simulink model "swing_up_sim"  (R2021a)
settings: Solver=VariableStepAuto  StartTime=0.0  StopTime=Inf  RelTol=1e-3
values from neighbouring files (symbols this model uses):
  alpha_0 = 0.0*pi    (= 0)    [swing_up_simulator.m]
  bp = 5e-5    (= 5e-05)    [qube2_rotpen_param.m]
  br = 1e-3    (= 0.001)    [qube2_rotpen_param.m]
  g = 9.81    [qube2_rotpen_param.m]
  Jp = mp*Lp^2/3    (= 0.000133128)    [qube2_rotpen_param.m]
  Jr = mr*r^2/3    (= 0.000228791666667)    [qube2_rotpen_param.m]
  l = Lp/2    (= 0.0645)    [qube2_rotpen_param.m]
  mp = 0.024    [qube2_rotpen_param.m]
  r = 0.085    [qube2_rotpen_param.m]
  tau_max = kt*10/Rm    (= 0.05)    [qube2_rotpen_param.m]
  thetadd_max = a_max/r    (= 72.8464760517)    [qube2_rotpen_param.m]
undefined symbols (not defined in the file or in its folder): rl
libraries: rllib x1
settings Model: Creator=willi  LastModifiedBy=willi

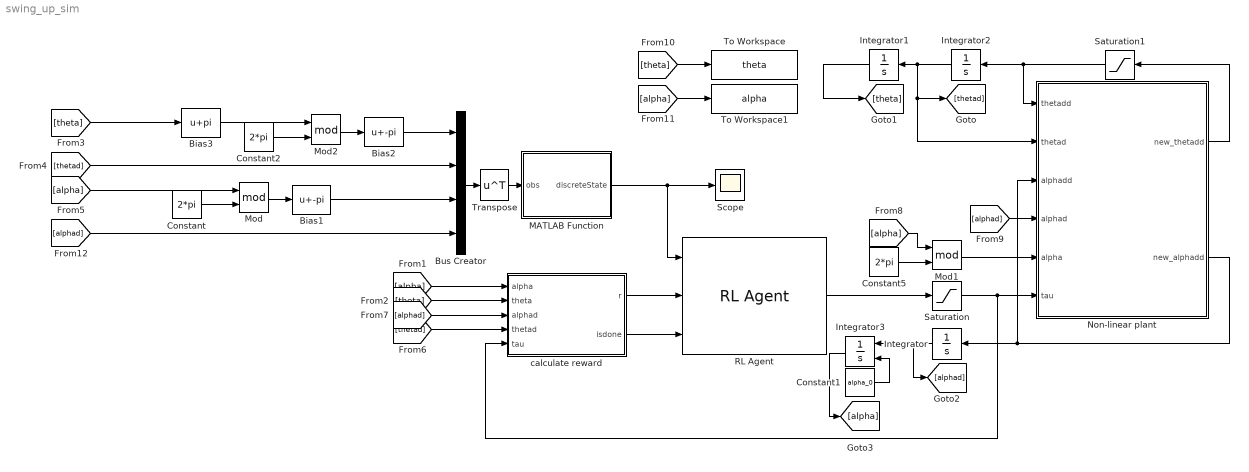
== system swing_up_sim ==
  Bias1 : Bias  Bias=-pi
  Bias2 : Bias  Bias=-pi
  Bias3 : Bias  Bias=pi
  Bus Creator : BusCreator  Inputs=4
  Constant : Constant  Value=2*pi
  Constant1 : Constant  Value=alpha_0
  Constant2 : Constant  Value=2*pi
  Constant5 : Constant  Value=2*pi
  Integrator : Integrator
  Integrator1 : Integrator
  Integrator2 : Integrator
  Integrator3 : Integrator  InitialConditionSource=external
  MATLAB Function : MATLAB Function  TreatAsAtomicUnit=on
  Mod : Math  Operator=mod  SaturateOnIntegerOverflow=on
  Mod1 : Math  Operator=mod  SaturateOnIntegerOverflow=on
  Mod2 : Math  Operator=mod  SaturateOnIntegerOverflow=on
  Non-linear plant : Subsystem
  RL Agent : rllib/RL Agent  Agent=rl.util.PolicyInstance.get('swing_up_sim/RL Agent')  ExternalActionAsInput=off  ProvideCumRwd=off  TreatAsDirectFeedthrough=on
  Saturation : Saturate  UpperLimit=tau_max  LowerLimit=-tau_max
  Saturation1 : Saturate  UpperLimit=thetadd_max  LowerLimit=-thetadd_max
  Scope : Scope
  To Workspace : ToWorkspace  VariableName=theta  SaveFormat=Timeseries  SampleTime=-1
  To Workspace1 : ToWorkspace  VariableName=alpha  SaveFormat=Timeseries  SampleTime=-1
  Transpose : Math  Operator=transpose  SaturateOnIntegerOverflow=on
  calculate reward : Subsystem
  wires:
  Non-linear plant/1(new_thetadd) -> Saturation1/1
  Non-linear plant/2(new_alphadd) -> Non-linear plant/3(alphadd), Integrator/1
  Constant1/1 -> Integrator3/2
  Constant5/1 -> Mod1/2
  Integrator1/1 -> [theta]
  Integrator3/1 -> [alpha]
  Integrator/1 -> [alphad], Integrator3/1
  Mod1/1 -> Non-linear plant/5(alpha)
  Integrator2/1 -> [thetad], Non-linear plant/2(thetad), Integrator1/1
  [alphad] -> Non-linear plant/4(alphad)
  [alpha] -> Mod1/1
  [alpha] -> To Workspace1/1
  [theta] -> To Workspace/1
  calculate reward/1(r) -> RL Agent/2
  RL Agent/1 -> Saturation/1
  Saturation/1 -> calculate reward/5(tau), Non-linear plant/6(tau)
  calculate reward/2(isdone) -> RL Agent/3
  [theta] -> calculate reward/2(theta)
  Saturation1/1 -> Integrator2/1, Non-linear plant/1(thetadd)
  [alpha] -> calculate reward/1(alpha)
  [alphad] -> calculate reward/3(alphad)
  [thetad] -> calculate reward/4(thetad)
  MATLAB Function/1(discreteState) -> Scope/1, RL Agent/1
  Bus Creator/1 -> Transpose/1
  Transpose/1 -> MATLAB Function/1(obs)
  Mod2/1 -> Bias2/1
  Mod/1 -> Bias1/1
  Bias3/1 -> Mod2/1
  Constant/1 -> Mod/2
  [alpha] -> Mod/1
  Constant2/1 -> Mod2/2
  Bias1/1 -> Bus Creator/3
  [alphad] -> Bus Creator/4
  [thetad] -> Bus Creator/2
  Bias2/1 -> Bus Creator/1
  [theta] -> Bias3/1

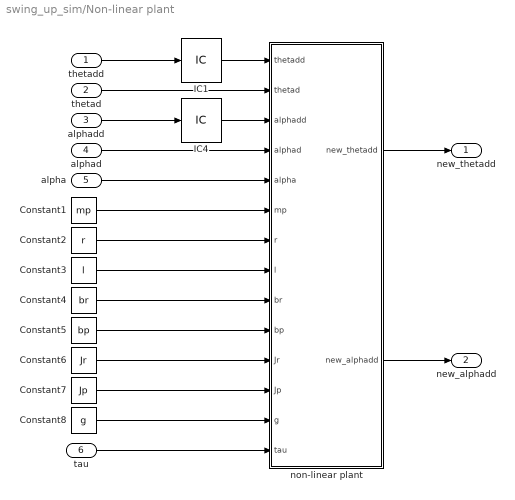
== system swing_up_sim/Non-linear plant ==
  thetadd : Inport
  thetad : Inport  Port=2
  alphadd : Inport  Port=3
  alphad : Inport  Port=4
  alpha : Inport  Port=5
  tau : Inport  Port=6
  Constant1 : Constant  Value=mp
  Constant2 : Constant  Value=r
  Constant3 : Constant  Value=l
  Constant4 : Constant  Value=br
  Constant5 : Constant  Value=bp
  Constant6 : Constant  Value=Jr
  Constant7 : Constant  Value=Jp
  Constant8 : Constant  Value=g
  IC1 : InitialCondition  Value=0
  IC4 : InitialCondition  Value=0
  non-linear plant : MATLAB Function  TreatAsAtomicUnit=on
  new_thetadd : Outport
  new_alphadd : Outport  Port=2
  wires:
  Constant3/1 -> non-linear plant/8(l)
  Constant2/1 -> non-linear plant/7(r)
  alphad/1 -> non-linear plant/4(alphad)
  non-linear plant/1(new_thetadd) -> new_thetadd/1
  alpha/1 -> non-linear plant/5(alpha)
  Constant1/1 -> non-linear plant/6(mp)
  Constant7/1 -> non-linear plant/12(Jp)
  non-linear plant/2(new_alphadd) -> new_alphadd/1
  Constant5/1 -> non-linear plant/10(bp)
  Constant4/1 -> non-linear plant/9(br)
  Constant8/1 -> non-linear plant/13(g)
  Constant6/1 -> non-linear plant/11(Jr)
  IC1/1 -> non-linear plant/1(thetadd)
  IC4/1 -> non-linear plant/3(alphadd)
  thetad/1 -> non-linear plant/2(thetad)
  thetadd/1 -> IC1/1
  alphadd/1 -> IC4/1
  tau/1 -> non-linear plant/14(tau)

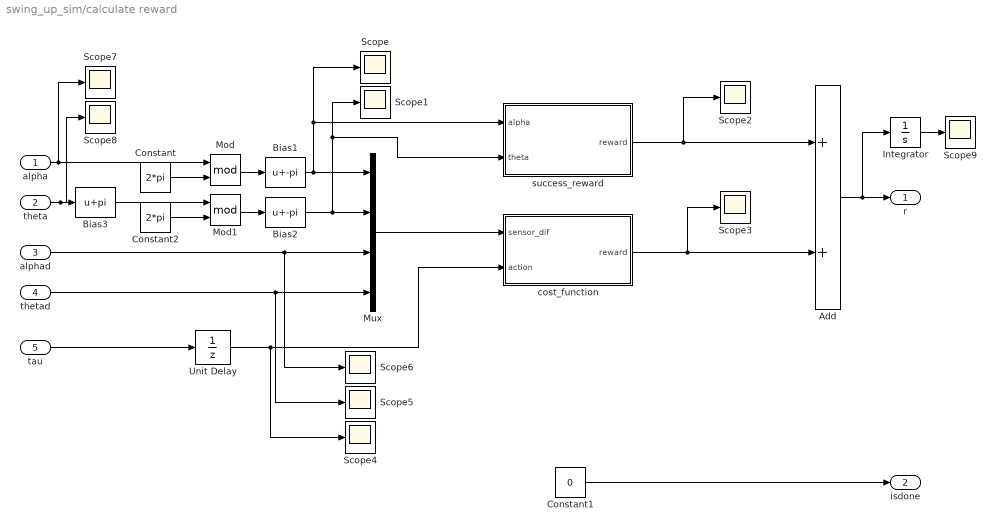
== system swing_up_sim/calculate reward ==
  alpha : Inport
  theta : Inport  Port=2
  alphad : Inport  Port=3
  thetad : Inport  Port=4
  tau : Inport  Port=5
  Add : Sum
  Bias1 : Bias  Bias=-pi
  Bias2 : Bias  Bias=-pi
  Bias3 : Bias  Bias=pi
  Constant : Constant  Value=2*pi
  Constant1 : Constant  Value=0
  Constant2 : Constant  Value=2*pi
  Integrator : Integrator
  Mod : Math  Operator=mod  SaturateOnIntegerOverflow=on
  Mod1 : Math  Operator=mod  SaturateOnIntegerOverflow=on
  Mux : Mux
  Scope{,1..9} (10 alike) : Scope
  Unit Delay : UnitDelay  SampleTime=-1  HasFrameUpgradeWarning=on
  cost_function : Subsystem
  success_reward : Subsystem
  r : Outport  VectorParamsAs1DForOutWhenUnconnected=off
  isdone : Outport  Port=2  VectorParamsAs1DForOutWhenUnconnected=off
  wires:
  tau/1 -> Unit Delay/1
  Constant/1 -> Mod/2
  Mod/1 -> Bias1/1
  alpha/1 -> Scope7/1, Mod/1
  Bias1/1 -> success_reward/1(alpha), Scope/1, Mux/1
  alphad/1 -> Scope6/1, Mux/3
  Unit Delay/1 -> Scope4/1, cost_function/2(action)
  Mux/1 -> cost_function/1(sensor_dif)
  success_reward/1(reward) -> Scope2/1, Add/1
  cost_function/1(reward) -> Scope3/1, Add/2
  Add/1 -> Integrator/1, r/1
  Constant1/1 -> isdone/1
  Constant2/1 -> Mod1/2
  theta/1 -> Scope8/1, Bias3/1
  Mod1/1 -> Bias2/1
  Bias2/1 -> Scope1/1, success_reward/2(theta), Mux/2
  Bias3/1 -> Mod1/1
  thetad/1 -> Scope5/1, Mux/4
  Integrator/1 -> Scope9/1

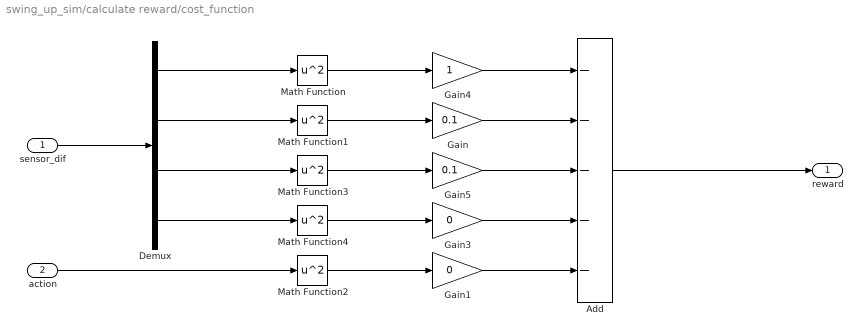
== system swing_up_sim/calculate reward/cost_function ==
  sensor_dif : Inport
  action : Inport  Port=2
  Add : Sum  Inputs=-----
  Demux : Demux
  Gain : Gain  Gain=0.1
  Gain1 : Gain  Gain=0
  Gain3 : Gain  Gain=0
  Gain4 : Gain
  Gain5 : Gain  Gain=0.1
  Math Function{,1..4} (5 alike) : Math  Operator=square  SaturateOnIntegerOverflow=on
  reward : Outport
  wires:
  Math Function4/1 -> Gain3/1
  Gain3/1 -> Add/4
  Gain1/1 -> Add/5
  Add/1 -> reward/1
  sensor_dif/1 -> Demux/1
  Demux/4 -> Math Function4/1
  Demux/3 -> Math Function3/1
  Demux/2 -> Math Function1/1
  Math Function1/1 -> Gain/1
  Math Function3/1 -> Gain5/1
  action/1 -> Math Function2/1
  Demux/1 -> Math Function/1
  Math Function/1 -> Gain4/1
  Math Function2/1 -> Gain1/1
  Gain4/1 -> Add/1
  Gain5/1 -> Add/3
  Gain/1 -> Add/2

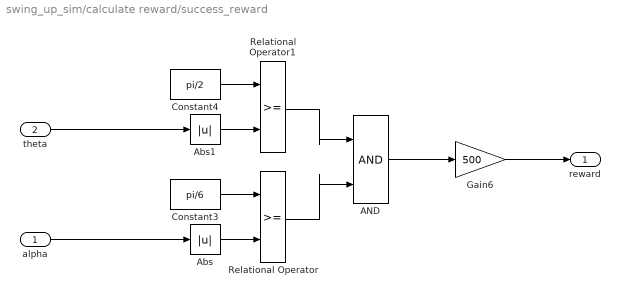
== system swing_up_sim/calculate reward/success_reward ==
  alpha : Inport
  theta : Inport  Port=2
  AND : Logic  IconShape=distinctive  AllPortsSameDT=off  OutDataTypeStr=boolean
  Abs : Abs
  Abs1 : Abs
  Constant3 : Constant  Value=pi/6
  Constant4 : Constant  Value=pi/2
  Gain6 : Gain  Gain=500
  Relational Operator : RelationalOperator  OutDataTypeStr=boolean  RndMeth=Simplest
  Relational Operator1 : RelationalOperator  OutDataTypeStr=boolean  RndMeth=Simplest
  reward : Outport
  wires:
  Gain6/1 -> reward/1
  Constant3/1 -> Relational Operator/1
  Abs/1 -> Relational Operator/2
  AND/1 -> Gain6/1
  Relational Operator/1 -> AND/2
  Abs1/1 -> Relational Operator1/2
  Constant4/1 -> Relational Operator1/1
  Relational Operator1/1 -> AND/1
  alpha/1 -> Abs/1
  theta/1 -> Abs1/1

== matlab function swing_up_sim/MATLAB Function ==
  data: obs input; discreteState output
function discreteState = fcn(obs)

obsHigh = [pi 50 pi 50];
obsLow = [-pi -50 -pi -50];

buckets = 4;
bucketSize = (obsHigh-obsLow)/buckets;

discreteState = floor((obs - obsLow)./bucketSize)+1;
discreteState = min(discreteState, buckets);
discreteState = max(discreteState, 1);

== matlab function swing_up_sim/Non-linear plant/non-linear plant ==
  data: thetadd input; thetad input; new_thetadd output; alphadd input; alphad input; alpha input; mp input; r input; l input; br input; bp input; Jr input; Jp input; g input; tau input; new_alphadd output
function [new_thetadd, new_alphadd]= fcn(thetadd, thetad, alphadd, alphad, alpha, mp, r, l, br, bp, Jr, Jp, g, tau)

new_alphadd = (-bp*alphad - mp*g*l*sin(alpha) + Jp*(thetad^2)*sin(alpha)*cos(alpha) - mp*l*r*thetadd*cos(alpha)) / Jp;
new_thetadd = (tau - br*thetad + mp*l*r*(alphad^2)*sin(alpha) - 2*Jp*alphad*thetad*sin(alpha)*cos(alpha) - mp*l*r*alphadd*cos(alpha)) / (Jr+Jp*(sin(alpha)^2));
